simulink model "eng_model"  (R2023a)
settings: Solver=VariableStepAuto  StartTime=0.0  StopTime=10  RelTol=1e-3
values from neighbouring files (symbols this model uses):
  C_m = 1.3    [CONSTANTS.m]
  C_w = 3.15    [CONSTANTS.m]
  J_eng = 7*10^(-6)    (= 7e-06)    [CONSTANTS.m]
  L_ov = 0.013    [CONSTANTS.m]
  L_ya = 0.0015    [CONSTANTS.m]
  R_ya = 8    [CONSTANTS.m]
settings Model: Creator=roma  LastModifiedBy=romav

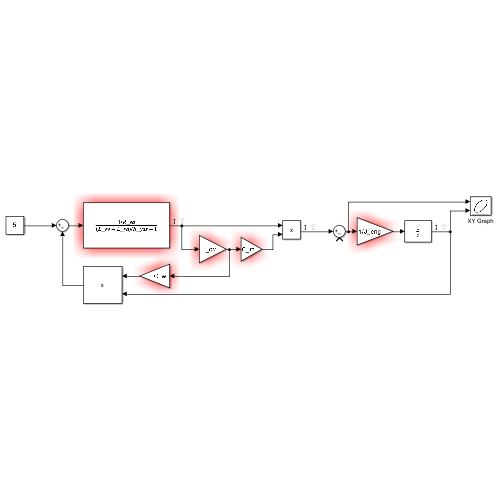
[thumbnail: Simulink's stored preview of the top-level diagram]
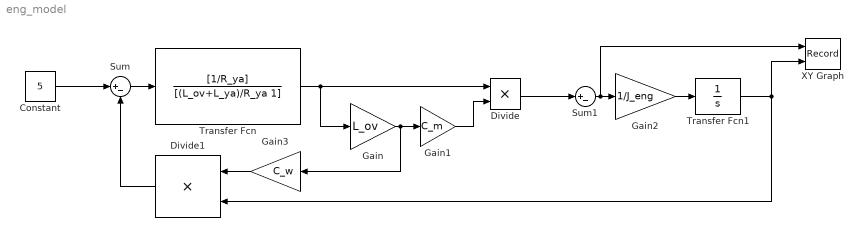
== system eng_model ==
  Constant : Constant  Value=5
  Divide : Product  Inputs=**
  Divide1 : Product  Inputs=**
  Gain : Gain  Gain=L_ov
  Gain1 : Gain  Gain=C_m
  Gain2 : Gain  Gain=1/J_eng
  Gain3 : Gain  Gain=C_w
  Sum : Sum  Inputs=|+-
  Sum1 : Sum  Inputs=|+-
  Transfer Fcn : TransferFcn  Numerator=[1/R_ya]  Denominator=[(L_ov+L_ya)/R_ya 1]
  Transfer Fcn1 : TransferFcn  Denominator=[1 0]
  XY Graph : Record  FileSettingsInternal="{\"entries\":[{\"content\":{\"excelSettings\":{\"content\":{},\"type\":\"Streamout.ExcelSettings\"}},\"type\":\"Streamout.FileSettingStorage\",\"uuid\":\"\"}],\"packageUris\":[\"http:\\/\\/schema.mathworks.com\\/mf0\\/streamout_blocks\\/R2020a\"],\"version\":\"1.0\"}"  Layout=[1 1]  SignalsInternal="{\"entries\":[{\"content\":{\"signals\":[{\"content\":{\"blockPath\":[],\"dimensions\":[1],\"domain\":\"\",\"lineColor\":\"#a2142f\",\"plots\":[1],\"port\":1,\"signalID\":8,\"signalName\":\"Sum1\"},\"type\":\"RecordBlkView.Signal\",\"uuid\":\"\"},{\"content\":{\"blockPath\":[],\"dimensions\":[1],\"domain\":\"\",\"lineColor\":\"#139fff\",\"plots\":[1],\"port\":2,\"signalID\":11,\"signalName\":\"Transfer Fcn1\"},\"type\":\"RecordBlkView.Signal\",\"uuid\":\"\"}]},\"type\":\"RecordBlkView.InputSignals\",\"uuid\":\"\"}],\"packageUris\":[\"http:\\/\\/schema.mathworks.com\\/mf0\\/streamout_blocks\\/R2020a\"],\"version\":\"1.0\"}"  VisualizationBindings="{\"xyplotplugin\":{\"info\":[{\"series\":[{\"bindingParametersList\":[{\"parameter\":\"X-Axis\",\"signalID\":8,\"signalName\":\"Sum1\"},{\"parameter\":\"Y-Axis\",\"signalID\":11,\"signalName\":\"Transfer Fcn1\"}],\"seriesID\":35389}],\"subplotID\":1}]}}"  CompatibilityTag=XY
  wires:
  Sum/1 -> Transfer Fcn/1
  Transfer Fcn/1 -> Gain/1, Divide/1
  Gain/1 -> Gain3/1, Gain1/1
  Gain1/1 -> Divide/2
  Divide/1 -> Sum1/1
  Gain2/1 -> Transfer Fcn1/1
  Transfer Fcn1/1 -> XY Graph/2, Divide1/2
  Gain3/1 -> Divide1/1
  Divide1/1 -> Sum/2
  Constant/1 -> Sum/1
  Sum1/1 -> XY Graph/1, Gain2/1
